simulink model "Controller2NonlinearSys"  (R2020b)
settings: Solver=VariableStepAuto  StartTime=0.0  StopTime=5  RelTol=1e-3
undefined symbols (not defined in the file): a, A, b, B, c, Cy_thetadot_phidot, Cy_thetadot_theta, d, e, F_thetadot_phidot, F_thetadot_theta, j, K_thetadot_phidot, K_thetadot_theta
settings Model: Creator=arthur  LastModifiedBy=arthur

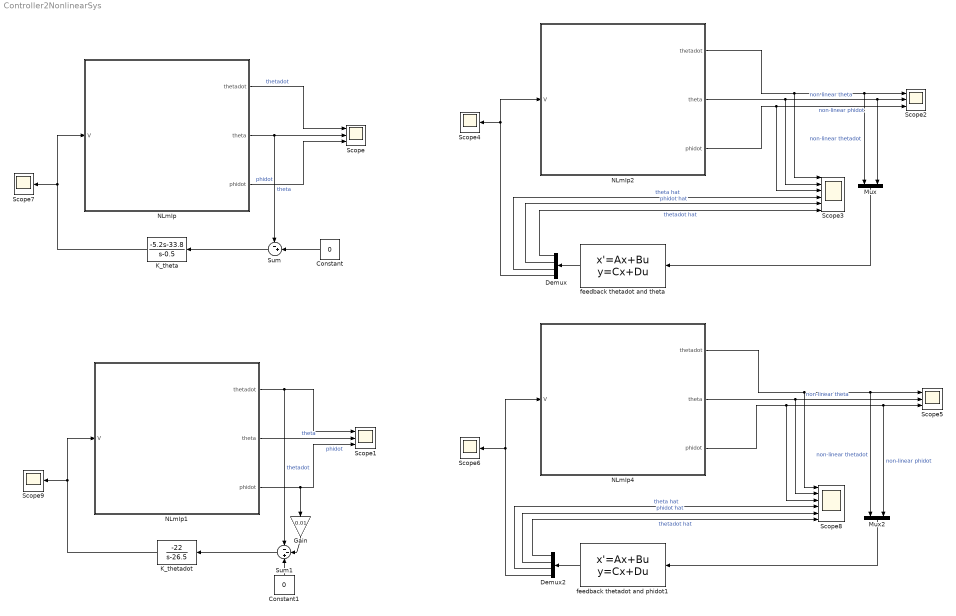
== system Controller2NonlinearSys ==
  Constant : Constant  Value=0
  Constant1 : Constant  Value=0
  Demux : Demux
  Demux2 : Demux
  Gain : Gain  Gain=0.01
  K_theta : TransferFcn  Numerator=[-5.2 -33.8]  Denominator=[1 -0.5]
  K_thetadot : TransferFcn  Numerator=[-22]  Denominator=[1 -26.5]
  Mux : Mux  Inputs=2
  Mux2 : Mux  Inputs=2
  NLmIp : Subsystem
  NLmIp1 : Subsystem
  NLmIp2 : Subsystem
  NLmIp4 : Subsystem
  Scope{,1..2,5} (4 alike) : Scope  NumInputPorts=3
  Scope3 : Scope  NumInputPorts=6
  Scope{4,6..7,9} (4 alike) : Scope
  Scope8 : Scope  NumInputPorts=6
  Sum : Sum  Inputs=-+|
  Sum1 : Sum  Inputs=--+
  feedback thetadot and phidot1 : StateSpace  A=A+B*K_thetadot_phidot+F_thetadot_phidot*Cy_thetadot_phidot  B=-F_thetadot_phidot  C=[eye(3);K_thetadot_phidot]  D=zeros(4,2)  InitialCondition=0
  feedback thetadot and theta : StateSpace  A=A+B*K_thetadot_theta+F_thetadot_theta*Cy_thetadot_theta  B=-F_thetadot_theta  C=[eye(3);K_thetadot_theta]  D=zeros(4,2)  InitialCondition=[0 0 0]
  wires:
  NLmIp/3(phidot) -> Scope/3  "phidot"
  NLmIp/2(theta) -> Scope/2, Sum/1  "theta"
  NLmIp/1(thetadot) -> Scope/1  "thetadot"
  K_theta/1 -> Scope7/1, NLmIp/1(V)
  Sum/1 -> K_theta/1
  Constant/1 -> Sum/2
  NLmIp1/1(thetadot) -> Sum1/1, Scope1/1  "thetadot"
  Sum1/1 -> K_thetadot/1
  NLmIp1/2(theta) -> Scope1/2  "theta"
  NLmIp1/3(phidot) -> Gain/1, Scope1/3  "phidot"
  K_thetadot/1 -> NLmIp1/1(V), Scope9/1
  Constant1/1 -> Sum1/3
  Gain/1 -> Sum1/2
  NLmIp2/2(theta) -> Scope2/2, Mux/2, Scope3/2  "non-linear theta"
  NLmIp2/1(thetadot) -> Scope2/1, Mux/1, Scope3/1  "non-linear thetadot"
  NLmIp2/3(phidot) -> Scope2/3, Scope3/3  "non-linear phidot"
  Mux/1 -> feedback thetadot and theta/1
  feedback thetadot and theta/1 -> Demux/1
  Demux/4 -> Scope4/1, NLmIp2/1(V)
  Demux/3 -> Scope3/4  "theta hat"
  Demux/2 -> Scope3/5  "phidot hat"
  Demux/1 -> Scope3/6  "thetadot hat"
  NLmIp4/3(phidot) -> Mux2/2, Scope5/3, Scope8/3  "non-linear phidot"
  NLmIp4/2(theta) -> Scope8/2, Scope5/2  "non-linear theta"
  NLmIp4/1(thetadot) -> Scope8/1, Scope5/1, Mux2/1  "non-linear thetadot"
  Mux2/1 -> feedback thetadot and phidot1/1
  feedback thetadot and phidot1/1 -> Demux2/1
  Demux2/4 -> NLmIp4/1(V), Scope6/1
  Demux2/3 -> Scope8/4  "theta hat"
  Demux2/2 -> Scope8/5  "phidot hat"
  Demux2/1 -> Scope8/6  "thetadot hat"

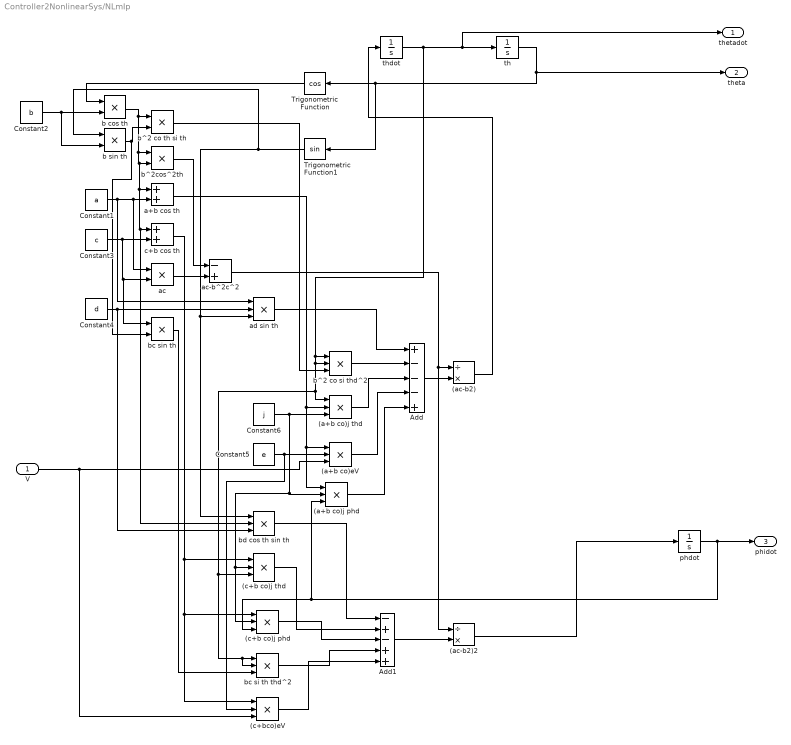
== system Controller2NonlinearSys/NLmIp ==
  V : Inport
  (a+b co)eV : Product  Inputs=3
  (a+b co)j phd : Product  Inputs=3
  (a+b co)j thd : Product  Inputs=3
  (ac-b2) : Product  Inputs=/*
  (ac-b2)2 : Product  Inputs=/*
  (c+b co)j phd : Product  Inputs=3
  (c+b co)j thd : Product  Inputs=3
  (c+bco)eV : Product  Inputs=3
  Add : Sum  Inputs=+---+
  Add1 : Sum  Inputs=-+-++
  Constant1 : Constant  Value=a
  Constant2 : Constant  Value=b
  Constant3 : Constant  Value=c
  Constant4 : Constant  Value=d
  Constant5 : Constant  Value=e
  Constant6 : Constant  Value=j
  Trigonometric Function : Trigonometry  Operator=cos
  Trigonometric Function1 : Trigonometry
  a+b cos th : Sum
  ac : Product
  ac-b^2c^2 : Sum  Inputs=-+
  ad sin th : Product  Inputs=3
  b cos th : Product
  b sin th : Product
  b^2 co si thd^2 : Product  Inputs=3
  b^2 co th si th : Product
  b^2cos^2th : Product
  bc si th thd^2 : Product  Inputs=3
  bc sin th : Product
  bd cos th sin th : Product  Inputs=3
  c+b cos th : Sum
  phdot : Integrator
  th : Integrator  InitialCondition=68*pi/180  ContinuousStateAttributes='theta'
  thdot : Integrator
  thetadot : Outport
  theta : Outport  Port=2
  phidot : Outport  Port=3
  wires:
  Trigonometric Function/1 -> b cos th/1
  (ac-b2)2/1 -> phdot/1
  V/1 -> (c+bco)eV/3, (a+b co)eV/3
  b^2 co th si th/1 -> b^2 co si thd^2/3
  ad sin th/1 -> Add/1
  c+b cos th/1 -> (c+bco)eV/1, (c+b co)j phd/1, (c+b co)j thd/1
  (c+b co)j phd/1 -> Add1/3
  Add/1 -> (ac-b2)/2
  (c+b co)j thd/1 -> Add1/2
  (a+b co)eV/1 -> Add/4
  b^2cos^2th/1 -> ac-b^2c^2/1
  b^2 co si thd^2/1 -> Add/2
  (ac-b2)/1 -> thdot/1
  (a+b co)j thd/1 -> Add/3
  b sin th/1 -> bc sin th/2, b^2 co th si th/2
  Constant5/1 -> (c+bco)eV/2, (a+b co)eV/2
  ac-b^2c^2/1 -> (ac-b2)2/1, (ac-b2)/1
  Constant3/1 -> bc sin th/1, ac/2, c+b cos th/2
  Constant6/1 -> (c+b co)j thd/2, (c+b co)j phd/2, (a+b co)j phd/2, (a+b co)j thd/3
  bd cos th sin th/1 -> Add1/1
  thdot/1 -> b^2 co si thd^2/1, b^2 co si thd^2/2, (c+b co)j thd/3, bc si th thd^2/2, bc si th thd^2/1, (a+b co)j thd/1, thetadot/1, th/1
  (a+b co)j phd/1 -> Add/5
  th/1 -> theta/1, Trigonometric Function1/1, Trigonometric Function/1
  Constant4/1 -> bd cos th sin th/3, ad sin th/2
  phdot/1 -> phidot/1, (c+b co)j phd/3, (a+b co)j phd/3
  Trigonometric Function1/1 -> b sin th/1, bd cos th sin th/1, ad sin th/3
  bc sin th/1 -> bc si th thd^2/3
  a+b cos th/1 -> (a+b co)j phd/1, (a+b co)eV/1, (a+b co)j thd/2
  Add1/1 -> (ac-b2)2/2
  ac/1 -> ac-b^2c^2/2
  bc si th thd^2/1 -> Add1/4
  (c+bco)eV/1 -> Add1/5
  b cos th/1 -> b^2 co th si th/1, bd cos th sin th/2, c+b cos th/1, a+b cos th/1, b^2cos^2th/2, b^2cos^2th/1
  Constant2/1 -> b sin th/2, b cos th/2
  Constant1/1 -> ad sin th/1, ac/1, a+b cos th/2

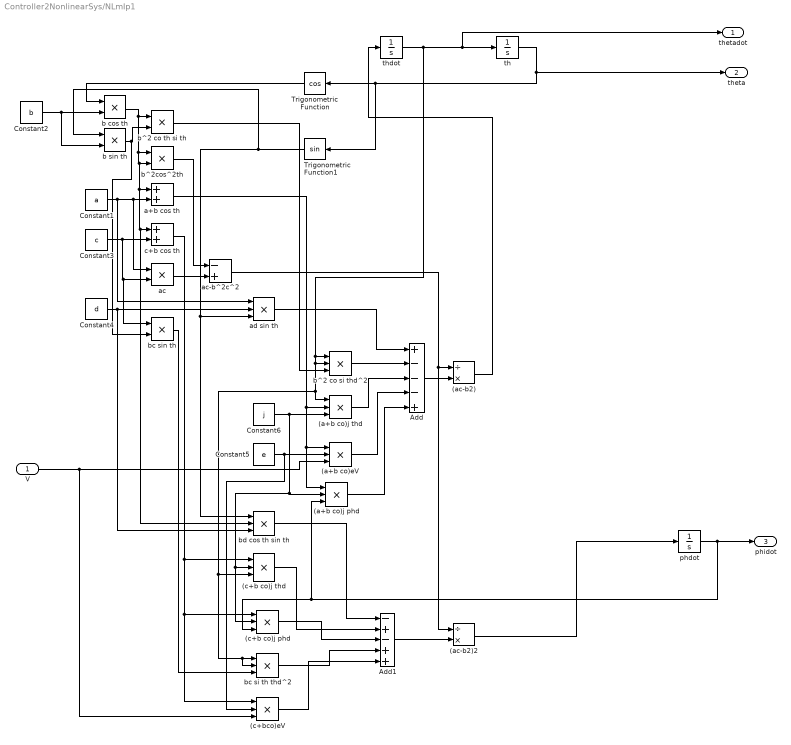
== system Controller2NonlinearSys/NLmIp1 ==
  V : Inport
  (a+b co)eV : Product  Inputs=3
  (a+b co)j phd : Product  Inputs=3
  (a+b co)j thd : Product  Inputs=3
  (ac-b2) : Product  Inputs=/*
  (ac-b2)2 : Product  Inputs=/*
  (c+b co)j phd : Product  Inputs=3
  (c+b co)j thd : Product  Inputs=3
  (c+bco)eV : Product  Inputs=3
  Add : Sum  Inputs=+---+
  Add1 : Sum  Inputs=-+-++
  Constant1 : Constant  Value=a
  Constant2 : Constant  Value=b
  Constant3 : Constant  Value=c
  Constant4 : Constant  Value=d
  Constant5 : Constant  Value=e
  Constant6 : Constant  Value=j
  Trigonometric Function : Trigonometry  Operator=cos
  Trigonometric Function1 : Trigonometry
  a+b cos th : Sum
  ac : Product
  ac-b^2c^2 : Sum  Inputs=-+
  ad sin th : Product  Inputs=3
  b cos th : Product
  b sin th : Product
  b^2 co si thd^2 : Product  Inputs=3
  b^2 co th si th : Product
  b^2cos^2th : Product
  bc si th thd^2 : Product  Inputs=3
  bc sin th : Product
  bd cos th sin th : Product  Inputs=3
  c+b cos th : Sum
  phdot : Integrator
  th : Integrator  InitialCondition=28*pi/180  ContinuousStateAttributes='theta'
  thdot : Integrator
  thetadot : Outport
  theta : Outport  Port=2
  phidot : Outport  Port=3
  wires:
  Trigonometric Function/1 -> b cos th/1
  (ac-b2)2/1 -> phdot/1
  V/1 -> (c+bco)eV/3, (a+b co)eV/3
  b^2 co th si th/1 -> b^2 co si thd^2/3
  ad sin th/1 -> Add/1
  c+b cos th/1 -> (c+bco)eV/1, (c+b co)j phd/1, (c+b co)j thd/1
  (c+b co)j phd/1 -> Add1/3
  Add/1 -> (ac-b2)/2
  (c+b co)j thd/1 -> Add1/2
  (a+b co)eV/1 -> Add/4
  b^2cos^2th/1 -> ac-b^2c^2/1
  b^2 co si thd^2/1 -> Add/2
  (ac-b2)/1 -> thdot/1
  (a+b co)j thd/1 -> Add/3
  b sin th/1 -> bc sin th/2, b^2 co th si th/2
  Constant5/1 -> (c+bco)eV/2, (a+b co)eV/2
  ac-b^2c^2/1 -> (ac-b2)2/1, (ac-b2)/1
  Constant3/1 -> bc sin th/1, ac/2, c+b cos th/2
  Constant6/1 -> (c+b co)j thd/2, (c+b co)j phd/2, (a+b co)j phd/2, (a+b co)j thd/3
  bd cos th sin th/1 -> Add1/1
  thdot/1 -> b^2 co si thd^2/1, b^2 co si thd^2/2, (c+b co)j thd/3, bc si th thd^2/2, bc si th thd^2/1, (a+b co)j thd/1, thetadot/1, th/1
  (a+b co)j phd/1 -> Add/5
  th/1 -> theta/1, Trigonometric Function1/1, Trigonometric Function/1
  Constant4/1 -> bd cos th sin th/3, ad sin th/2
  phdot/1 -> phidot/1, (c+b co)j phd/3, (a+b co)j phd/3
  Trigonometric Function1/1 -> b sin th/1, bd cos th sin th/1, ad sin th/3
  bc sin th/1 -> bc si th thd^2/3
  a+b cos th/1 -> (a+b co)j phd/1, (a+b co)eV/1, (a+b co)j thd/2
  Add1/1 -> (ac-b2)2/2
  ac/1 -> ac-b^2c^2/2
  bc si th thd^2/1 -> Add1/4
  (c+bco)eV/1 -> Add1/5
  b cos th/1 -> b^2 co th si th/1, bd cos th sin th/2, c+b cos th/1, a+b cos th/1, b^2cos^2th/2, b^2cos^2th/1
  Constant2/1 -> b sin th/2, b cos th/2
  Constant1/1 -> ad sin th/1, ac/1, a+b cos th/2

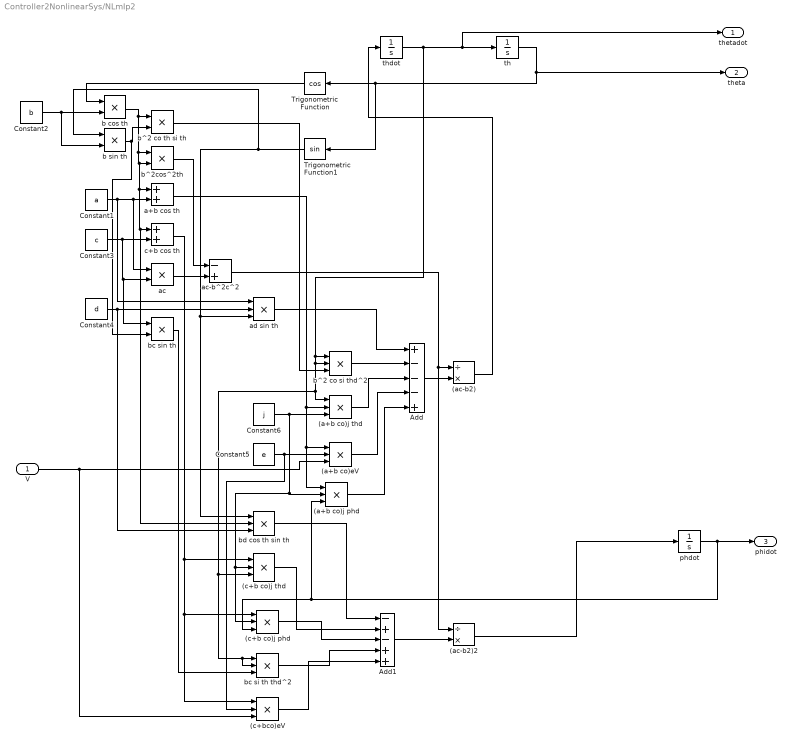
== system Controller2NonlinearSys/NLmIp2 ==
  V : Inport
  (a+b co)eV : Product  Inputs=3
  (a+b co)j phd : Product  Inputs=3
  (a+b co)j thd : Product  Inputs=3
  (ac-b2) : Product  Inputs=/*
  (ac-b2)2 : Product  Inputs=/*
  (c+b co)j phd : Product  Inputs=3
  (c+b co)j thd : Product  Inputs=3
  (c+bco)eV : Product  Inputs=3
  Add : Sum  Inputs=+---+
  Add1 : Sum  Inputs=-+-++
  Constant1 : Constant  Value=a
  Constant2 : Constant  Value=b
  Constant3 : Constant  Value=c
  Constant4 : Constant  Value=d
  Constant5 : Constant  Value=e
  Constant6 : Constant  Value=j
  Trigonometric Function : Trigonometry  Operator=cos
  Trigonometric Function1 : Trigonometry
  a+b cos th : Sum
  ac : Product
  ac-b^2c^2 : Sum  Inputs=-+
  ad sin th : Product  Inputs=3
  b cos th : Product
  b sin th : Product
  b^2 co si thd^2 : Product  Inputs=3
  b^2 co th si th : Product
  b^2cos^2th : Product
  bc si th thd^2 : Product  Inputs=3
  bc sin th : Product
  bd cos th sin th : Product  Inputs=3
  c+b cos th : Sum
  phdot : Integrator
  th : Integrator  InitialCondition=69*pi/180  ContinuousStateAttributes='theta'
  thdot : Integrator
  thetadot : Outport
  theta : Outport  Port=2
  phidot : Outport  Port=3
  wires:
  Trigonometric Function/1 -> b cos th/1
  (ac-b2)2/1 -> phdot/1
  V/1 -> (c+bco)eV/3, (a+b co)eV/3
  b^2 co th si th/1 -> b^2 co si thd^2/3
  ad sin th/1 -> Add/1
  c+b cos th/1 -> (c+bco)eV/1, (c+b co)j phd/1, (c+b co)j thd/1
  (c+b co)j phd/1 -> Add1/3
  Add/1 -> (ac-b2)/2
  (c+b co)j thd/1 -> Add1/2
  (a+b co)eV/1 -> Add/4
  b^2cos^2th/1 -> ac-b^2c^2/1
  b^2 co si thd^2/1 -> Add/2
  (ac-b2)/1 -> thdot/1
  (a+b co)j thd/1 -> Add/3
  b sin th/1 -> bc sin th/2, b^2 co th si th/2
  Constant5/1 -> (c+bco)eV/2, (a+b co)eV/2
  ac-b^2c^2/1 -> (ac-b2)2/1, (ac-b2)/1
  Constant3/1 -> bc sin th/1, ac/2, c+b cos th/2
  Constant6/1 -> (c+b co)j thd/2, (c+b co)j phd/2, (a+b co)j phd/2, (a+b co)j thd/3
  bd cos th sin th/1 -> Add1/1
  thdot/1 -> b^2 co si thd^2/1, b^2 co si thd^2/2, (c+b co)j thd/3, bc si th thd^2/2, bc si th thd^2/1, (a+b co)j thd/1, thetadot/1, th/1
  (a+b co)j phd/1 -> Add/5
  th/1 -> theta/1, Trigonometric Function1/1, Trigonometric Function/1
  Constant4/1 -> bd cos th sin th/3, ad sin th/2
  phdot/1 -> phidot/1, (c+b co)j phd/3, (a+b co)j phd/3
  Trigonometric Function1/1 -> b sin th/1, bd cos th sin th/1, ad sin th/3
  bc sin th/1 -> bc si th thd^2/3
  a+b cos th/1 -> (a+b co)j phd/1, (a+b co)eV/1, (a+b co)j thd/2
  Add1/1 -> (ac-b2)2/2
  ac/1 -> ac-b^2c^2/2
  bc si th thd^2/1 -> Add1/4
  (c+bco)eV/1 -> Add1/5
  b cos th/1 -> b^2 co th si th/1, bd cos th sin th/2, c+b cos th/1, a+b cos th/1, b^2cos^2th/2, b^2cos^2th/1
  Constant2/1 -> b sin th/2, b cos th/2
  Constant1/1 -> ad sin th/1, ac/1, a+b cos th/2

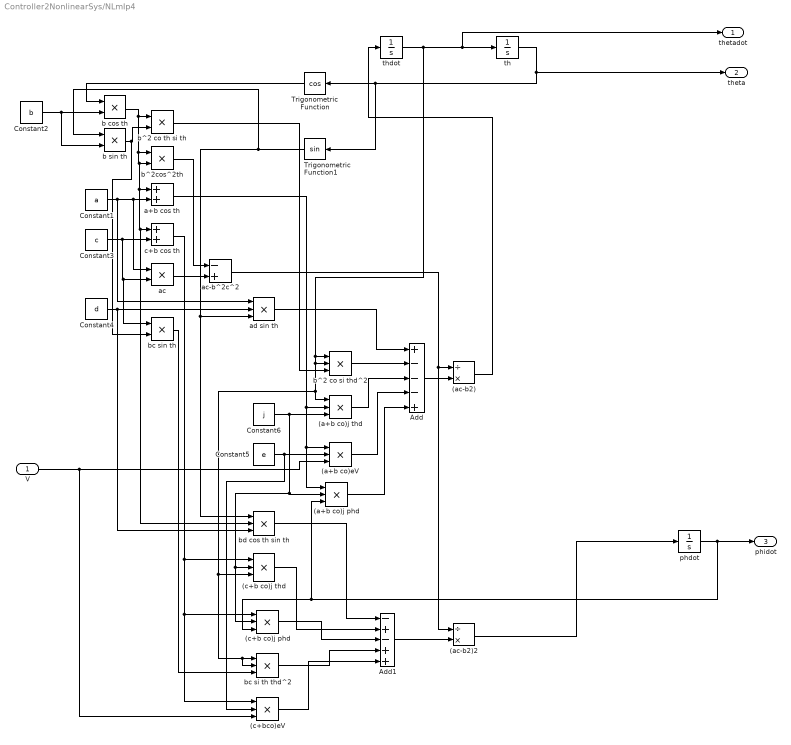
== system Controller2NonlinearSys/NLmIp4 ==
  V : Inport
  (a+b co)eV : Product  Inputs=3
  (a+b co)j phd : Product  Inputs=3
  (a+b co)j thd : Product  Inputs=3
  (ac-b2) : Product  Inputs=/*
  (ac-b2)2 : Product  Inputs=/*
  (c+b co)j phd : Product  Inputs=3
  (c+b co)j thd : Product  Inputs=3
  (c+bco)eV : Product  Inputs=3
  Add : Sum  Inputs=+---+
  Add1 : Sum  Inputs=-+-++
  Constant1 : Constant  Value=a
  Constant2 : Constant  Value=b
  Constant3 : Constant  Value=c
  Constant4 : Constant  Value=d
  Constant5 : Constant  Value=e
  Constant6 : Constant  Value=j
  Trigonometric Function : Trigonometry  Operator=cos
  Trigonometric Function1 : Trigonometry
  a+b cos th : Sum
  ac : Product
  ac-b^2c^2 : Sum  Inputs=-+
  ad sin th : Product  Inputs=3
  b cos th : Product
  b sin th : Product
  b^2 co si thd^2 : Product  Inputs=3
  b^2 co th si th : Product
  b^2cos^2th : Product
  bc si th thd^2 : Product  Inputs=3
  bc sin th : Product
  bd cos th sin th : Product  Inputs=3
  c+b cos th : Sum
  phdot : Integrator
  th : Integrator  InitialCondition=53*pi/180  ContinuousStateAttributes='theta'
  thdot : Integrator
  thetadot : Outport
  theta : Outport  Port=2
  phidot : Outport  Port=3
  wires:
  Trigonometric Function/1 -> b cos th/1
  (ac-b2)2/1 -> phdot/1
  V/1 -> (c+bco)eV/3, (a+b co)eV/3
  b^2 co th si th/1 -> b^2 co si thd^2/3
  ad sin th/1 -> Add/1
  c+b cos th/1 -> (c+bco)eV/1, (c+b co)j phd/1, (c+b co)j thd/1
  (c+b co)j phd/1 -> Add1/3
  Add/1 -> (ac-b2)/2
  (c+b co)j thd/1 -> Add1/2
  (a+b co)eV/1 -> Add/4
  b^2cos^2th/1 -> ac-b^2c^2/1
  b^2 co si thd^2/1 -> Add/2
  (ac-b2)/1 -> thdot/1
  (a+b co)j thd/1 -> Add/3
  b sin th/1 -> bc sin th/2, b^2 co th si th/2
  Constant5/1 -> (c+bco)eV/2, (a+b co)eV/2
  ac-b^2c^2/1 -> (ac-b2)2/1, (ac-b2)/1
  Constant3/1 -> bc sin th/1, ac/2, c+b cos th/2
  Constant6/1 -> (c+b co)j thd/2, (c+b co)j phd/2, (a+b co)j phd/2, (a+b co)j thd/3
  bd cos th sin th/1 -> Add1/1
  thdot/1 -> b^2 co si thd^2/1, b^2 co si thd^2/2, (c+b co)j thd/3, bc si th thd^2/2, bc si th thd^2/1, (a+b co)j thd/1, thetadot/1, th/1
  (a+b co)j phd/1 -> Add/5
  th/1 -> theta/1, Trigonometric Function1/1, Trigonometric Function/1
  Constant4/1 -> bd cos th sin th/3, ad sin th/2
  phdot/1 -> phidot/1, (c+b co)j phd/3, (a+b co)j phd/3
  Trigonometric Function1/1 -> b sin th/1, bd cos th sin th/1, ad sin th/3
  bc sin th/1 -> bc si th thd^2/3
  a+b cos th/1 -> (a+b co)j phd/1, (a+b co)eV/1, (a+b co)j thd/2
  Add1/1 -> (ac-b2)2/2
  ac/1 -> ac-b^2c^2/2
  bc si th thd^2/1 -> Add1/4
  (c+bco)eV/1 -> Add1/5
  b cos th/1 -> b^2 co th si th/1, bd cos th sin th/2, c+b cos th/1, a+b cos th/1, b^2cos^2th/2, b^2cos^2th/1
  Constant2/1 -> b sin th/2, b cos th/2
  Constant1/1 -> ad sin th/1, ac/1, a+b cos th/2
